simulink library "raspberrypi_drivers"  (R2014a)
settings: Solver=ode45  StartTime=0.0  StopTime=10.0  FixedStep=0.01  RelTol=1e-3
settings Model: Creator=odufour  LastModifiedBy=odufour

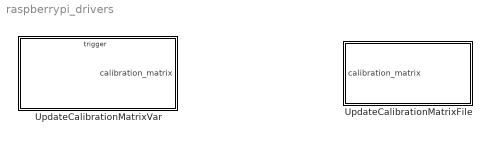
== system raspberrypi_drivers ==
  UpdateCalibrationMatrixFile : Subsystem
  UpdateCalibrationMatrixVar : Subsystem

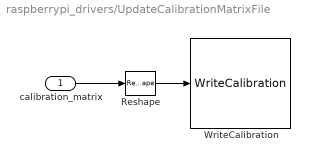
== system raspberrypi_drivers/UpdateCalibrationMatrixFile ==
  calibration_matrix : Inport
  Reshape : Reshape
  WriteCalibration : S-Function  FunctionName=WriteCalibration  EnableBusSupport=off
  wires:
  calibration_matrix/1 -> Reshape/1
  Reshape/1 -> WriteCalibration/1

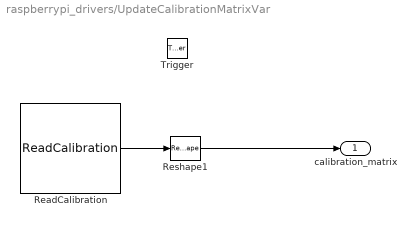
== system raspberrypi_drivers/UpdateCalibrationMatrixVar ==
  Trigger : TriggerPort  PortDimensions=1
  ReadCalibration : S-Function  FunctionName=ReadCalibration  EnableBusSupport=off
  Reshape1 : Reshape  OutputDimensionality=Customize  OutputDimensions=[3,3]
  calibration_matrix : Outport
  wires:
  Reshape1/1 -> calibration_matrix/1
  ReadCalibration/1 -> Reshape1/1
